simulink model "Controlador_Otimo_Aero"  (R2018a)
settings: Solver=FixedStepAuto  StartTime=0.0  StopTime=70  RelTol=1e-3  EnableMultiTasking=on
values from neighbouring files (symbols this model uses):
  C = [1 0 0 0 ... (first row only)    [Dados.m]    (also in Dados_correct.m; Function_ARE.m = D; teste.m = D)
  K1_30 = Kpi30(:,1:4)    [Dados_correct.m]
  K2_30 = Kpi30(:,5:6)    [Dados_correct.m]
  Pphi = polyfit(phi,y_phi,2)    [Pot.m]
  Pteta = polyfit(teta,y_teta,2)    [Pot.m]
undefined symbols (not defined in the file or in its folder): DiscIntNeverNeededParam, K1_130, K1_150, K1_90, K2_130, K2_150, K2_90, sigbuilder_block
libraries: arduinolib x4, simulink x2
settings Model: SimulationMode=external  ExtModeTrigDuration=2  Creator=stayn  LastModifiedBy=stayn
settings OptimizationCC: EnhancedBackFolding=on  PassReuseOutputArgsAs=Individual arguments  MaxStackSize=64  OptimizeBlockOrder=speed  DifferentSizesBufferReuse=on  OptimizationCustomize=off
settings DebuggingCC: ParameterTunabilityLossMsg=error
settings HardwareCC: ProdBitPerInt=16  ProdBitPerPointer=16  ProdBitPerSizeT=16  ProdBitPerPtrDiffT=16  ProdLargestAtomicFloat=None  ProdWordSize=8  ProdHWDeviceType=Atmel->AVR
settings SFSimCC: MATLABDynamicMemAlloc=off
settings RTWCC: SystemTargetFile=ert.tlc  HardwareBoard=Arduino Mega 2560  TLCOptions=-aInlineSetEventsForThisBaseRateFcn=TLC_FALSE -aSuppressMultiTaskScheduler=TLC_FALSE -aRateBasedStepFcn=1  TemplateMakefile=ert_default_tmf  GenerateReport=on  Toolchain=Arduino AVR  BuildConfiguration=Faster Runs  IncludeHyperlinkInReport=on  LaunchReport=on  GenerateTraceInfo=on  GenerateTraceReport=on  GenerateTraceReportSl=on  GenerateTraceReportSf=on  GenerateTraceReportEml=on
settings CodeAppCC: ForceParamTrailComments=on  IgnoreCustomStorageClasses=off  OperatorAnnotations=on  SimulinkDataObjDesc=on  SFDataObjDesc=on  InsertBlockDesc=on
settings ERTTargetCC: SupportContinuousTime=on  SupportVariableSizeSignals=on

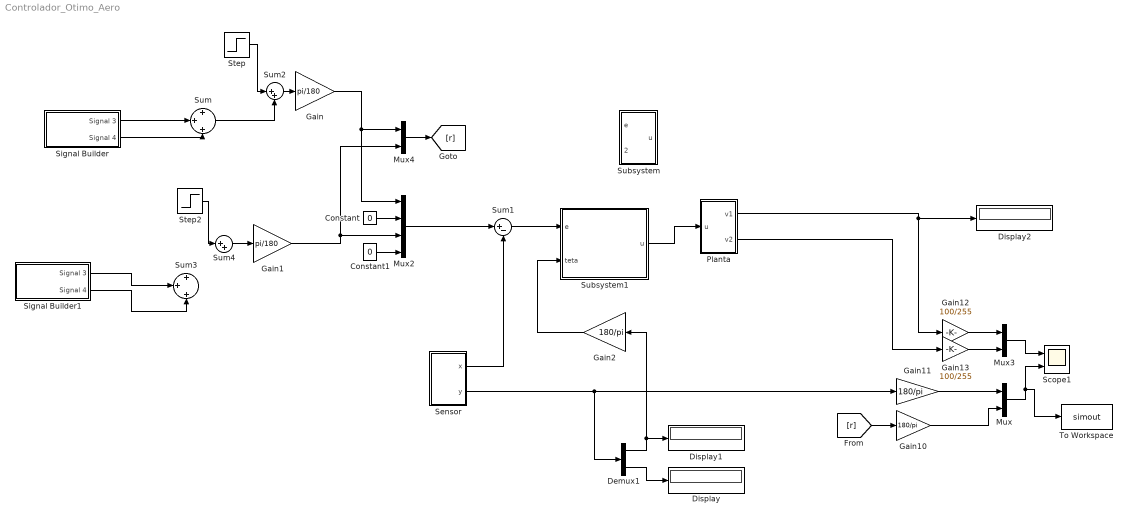
== system Controlador_Otimo_Aero ==
  Constant : Constant  Value=0
  Constant1 : Constant  Value=0
  Demux1 : Demux  Outputs=2
  Display : Display
  Display1 : Display
  Display2 : Display
  Gain : Gain  Gain=pi/180
  Gain1 : Gain  Gain=pi/180
  Gain10 : Gain  Gain=180/pi
  Gain11 : Gain  Gain=180/pi
  Gain12 : Gain  Gain=100/255
  Gain13 : Gain  Gain=100/255
  Gain2 : Gain  Gain=180/pi
  Mux : Mux  Inputs=2
  Mux2 : Mux
  Mux3 : Mux  Inputs=2
  Mux4 : Mux  Inputs=2
  Planta : Subsystem
  Scope1 : Scope  NumInputPorts=2
  Sensor : Subsystem
  Signal Builder : Subsystem  Tag=STV Subsys  LoadFcn=sigbuilder_block('load');  StartFcn=sigbuilder_block('start');  StopFcn=sigbuilder_block('stop');  ClipboardFcn=sigbuilder_block('clipboard');  mask(Sigbuilder block){tuvar=[0:10]}
      mask help: Simulink:masks:SigbuilderBlock_MD
      mask init:
      | if ~strcmp(get_param(bdroot(gcbh),'SimulationStatus'),'stopped') tuvar = sigbuilder_block('maskInit'); end
      settings: CopyFcn=sigbuilder_block('copy');  DeleteFcn=sigbuilder_block('delete');  ModelCloseFcn=sigbuilder_block('modelClose');  PreSaveFcn=sigbuilder_block('preSave');  PauseFcn=sigbuilder_block('pause');  ContinueFcn=sigbuilder_block('continue');  NameChangeFcn=sigbuilder_block('namechange');  OpenFcn=sigbuilder_block('open',[6 30 1012.5 447.75 ]);  CloseFcn=sigbuilder_block('close');
      mask Display: plot(0, 0, 100, 100,[2, 2, 32, 32, 2], [68, 8, 8, 68, 68],[32, 2], [38, 38], [32, 19, 2],[53, 60, 44], [32, 17, 17, 2],[16, 16, 31, 31]);txt = getActiveGroup(gcbh);text(2, 100, txt,'verticalAlignment', 'top');
  Signal Builder1 : Subsystem  Tag=STV Subsys  LoadFcn=sigbuilder_block('load');  StartFcn=sigbuilder_block('start');  StopFcn=sigbuilder_block('stop');  ClipboardFcn=sigbuilder_block('clipboard');  mask(Sigbuilder block){tuvar=[0:10]}
      mask help: Simulink:masks:SigbuilderBlock_MD
      mask init:
      | if ~strcmp(get_param(bdroot(gcbh),'SimulationStatus'),'stopped') tuvar = sigbuilder_block('maskInit'); end
      settings: CopyFcn=sigbuilder_block('copy');  DeleteFcn=sigbuilder_block('delete');  ModelCloseFcn=sigbuilder_block('modelClose');  PreSaveFcn=sigbuilder_block('preSave');  PauseFcn=sigbuilder_block('pause');  ContinueFcn=sigbuilder_block('continue');  NameChangeFcn=sigbuilder_block('namechange');  OpenFcn=sigbuilder_block('open',[6 30 1006.5 447.75 ]);  CloseFcn=sigbuilder_block('close');
      mask Display: plot(0, 0, 100, 100,[2, 2, 32, 32, 2], [68, 8, 8, 68, 68],[32, 2], [38, 38], [32, 19, 2],[53, 60, 44], [32, 17, 17, 2],[16, 16, 31, 31]);txt = getActiveGroup(gcbh);text(2, 100, txt,'verticalAlignment', 'top');
  Step : Step  Time=0  After=110  SampleTime=0
  Step2 : Step  After=25  SampleTime=0
  Subsystem : Subsystem
  Subsystem1 : Subsystem
  Sum : Sum  Inputs=+|+|+
  Sum1 : Sum  Inputs=|+-
  Sum2 : Sum  Inputs=|++
  Sum3 : Sum  Inputs=+|+|+
  Sum4 : Sum  Inputs=|++
  To Workspace : ToWorkspace  VariableName=simout  SampleTime=-1
      settings: Save2DSignal=2-D array (concatenate along first dimension)
  wires:
  Mux3/1 -> Scope1/1
  Mux/1 -> To Workspace/1, Scope1/2
  [r] -> Gain10/1
  Gain10/1 -> Mux/2
  Gain11/1 -> Mux/1
  Gain12/1 -> Mux3/1
  Gain13/1 -> Mux3/2
  Sum1/1 -> Subsystem1/1(e)
  Sensor/1("x ") -> Sum1/2
  Sensor/2(y) -> Demux1/1, Gain11/1
  Demux1/2 -> Display/1
  Subsystem1/1(u) -> Planta/1(u)
  Planta/1(v1) -> Display2/1, Gain12/1
  Planta/2("v2 ") -> Gain13/1
  Demux1/1 -> Display1/1, Gain2/1
  Gain2/1 -> Subsystem1/2(teta)
  Step2/1 -> Sum4/1
  Sum/1 -> Sum2/2
  Signal Builder1/1(Signal 3) -> Sum3/2
  Sum4/1 -> Gain1/1
  Signal Builder/1(Signal 3) -> Sum/2
  Signal Builder1/2(Signal 4) -> Sum3/3
  Constant1/1 -> Mux2/4
  Constant/1 -> Mux2/2
  Mux2/1 -> Sum1/1
  Mux4/1 -> [r]
  Gain1/1 -> Mux4/2, Mux2/3
  Step/1 -> Sum2/1
  Sum2/1 -> Gain/1
  Gain/1 -> Mux2/1, Mux4/1
  Signal Builder/2(Signal 4) -> Sum/3

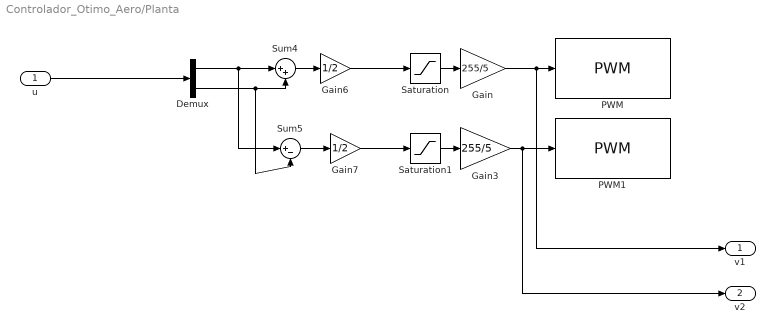
== system Controlador_Otimo_Aero/Planta ==
  u : Inport
  Demux : Demux  Outputs=2
  Gain : Gain  Gain=255/5
  Gain3 : Gain  Gain=255/5
  Gain6 : Gain  Gain=1/2
  Gain7 : Gain  Gain=1/2
  PWM : arduinolib/PWM  pinNumber=9  EnableInputFrequency=off  InitialFrequency=2000  InitialDutyCycle=0  NotificationType=None  blockPlatform=arduino
  PWM1 : arduinolib/PWM  pinNumber=8  EnableInputFrequency=off  InitialFrequency=2000  InitialDutyCycle=0  NotificationType=None  blockPlatform=arduino
  Saturation : Saturate  UpperLimit=5  LowerLimit=0
  Saturation1 : Saturate  UpperLimit=5  LowerLimit=0
  Sum4 : Sum  Inputs=|++
  Sum5 : Sum  Inputs=|+-
  v1 : Outport
  "v2 " : Outport  Port=2
  wires:
  Sum4/1 -> Gain6/1
  Demux/1 -> Sum5/1, Sum4/1
  Saturation1/1 -> Gain3/1
  Gain7/1 -> Saturation1/1
  Demux/2 -> Sum5/2, Sum4/2
  Gain/1 -> PWM/1, v1/1
  Saturation/1 -> Gain/1
  Gain6/1 -> Saturation/1
  Gain3/1 -> PWM1/1, "v2 "/1
  Sum5/1 -> Gain7/1
  u/1 -> Demux/1

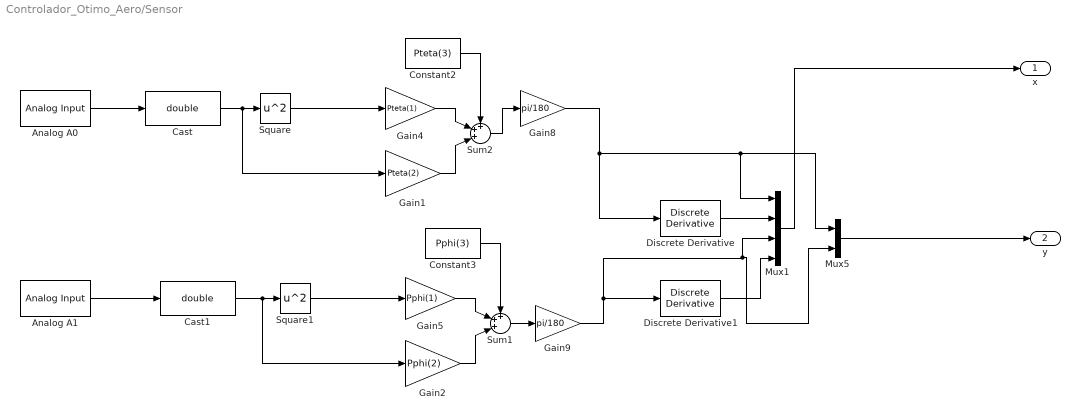
== system Controlador_Otimo_Aero/Sensor ==
  Analog A0 : arduinolib/Analog Input  pinNumber=0  ReadResultsOnly=off  ConversionTriggerSource=Software  ExternalTriggerType=uint32(0)  OutputDataType=uint16  EnableConversionCompleteNotify=off  EnableOuputStatus=off  SampleTime=-1  blockPlatform=arduino
  Analog A1 : arduinolib/Analog Input  pinNumber=1  ReadResultsOnly=off  ConversionTriggerSource=Software  ExternalTriggerType=uint32(0)  OutputDataType=uint16  EnableConversionCompleteNotify=off  EnableOuputStatus=off  SampleTime=-1  blockPlatform=arduino
  Cast : DataTypeConversion  OutDataTypeStr=double
  Cast1 : DataTypeConversion  OutDataTypeStr=double
  Constant2 : Constant  Value=Pteta(3)
  Constant3 : Constant  Value=Pphi(3)
  Discrete Derivative : simulink/Discrete/Discrete Derivative  gainval=1.0  ICPrevScaledInput=0.0  OutMin=[]  OutMax=[]  OutDataType=fixdt(1, 16)  OutScaling=2^-10  DoSatur=off
  Discrete Derivative1 : simulink/Discrete/Discrete Derivative  gainval=1.0  ICPrevScaledInput=0.0  OutMin=[]  OutMax=[]  OutDataType=fixdt(1, 16)  OutScaling=2^-10  DoSatur=off
  Gain1 : Gain  Gain=Pteta(2)
  Gain2 : Gain  Gain=Pphi(2)
  Gain4 : Gain  Gain=Pteta(1)
  Gain5 : Gain  Gain=Pphi(1)
  Gain8 : Gain  Gain=pi/180
  Gain9 : Gain  Gain=pi/180
  Mux1 : Mux
  Mux5 : Mux  Inputs=2
  Square : Math  Operator=square  SaturateOnIntegerOverflow=on
  Square1 : Math  Operator=square  SaturateOnIntegerOverflow=on
  Sum1 : Sum  Inputs=+++|
  Sum2 : Sum  Inputs=+++|
  "x " : Outport
  y : Outport  Port=2
  wires:
  Mux5/1 -> y/1
  Gain9/1 -> Discrete Derivative1/1, Mux5/2, Mux1/3
  Gain8/1 -> Mux5/1, Mux1/1, Discrete Derivative/1
  Discrete Derivative1/1 -> Mux1/4
  Mux1/1 -> "x "/1
  Discrete Derivative/1 -> Mux1/2
  Cast1/1 -> Gain2/1, Square1/1
  Square1/1 -> Gain5/1
  Sum1/1 -> Gain9/1
  Gain5/1 -> Sum1/2
  Constant3/1 -> Sum1/1
  Gain1/1 -> Sum2/3
  Analog A1/1 -> Cast1/1
  Analog A0/1 -> Cast/1
  Gain4/1 -> Sum2/2
  Cast/1 -> Gain1/1, Square/1
  Constant2/1 -> Sum2/1
  Sum2/1 -> Gain8/1
  Square/1 -> Gain4/1
  Gain2/1 -> Sum1/3

== system Controlador_Otimo_Aero/Signal Builder ==
  Demux : Demux  Tag=STV Demux  Outputs=2
  FromWs : FromWorkspace  Tag=STV FromWs  VariableName=tuvar  SampleTime=0
      SigBuilderData=|
      | common.afterFinalStr = 'Extrapolate'
      | common.sampleTime = 0
      | dataSet.timeRange = [0 100]
      | dataSet.name = 'Group 1'
      | sbobj.Groups.Name = 'Group 1'
      | sbobj.Groups.Signals(1).Name = 'Signal 3'
      | sbobj.Groups.Signals(1).XData = [0 15.1 15.1 30 30 100]
      | sbobj.Groups.Signals(1).YData = [0 0 40 40 0 0]
      | sbobj.Groups.Signals(2).Name = 'Signal 4'
      | sbobj.Groups.Signals(2).XData = [0 45 45 60 60 100]
      | sbobj.Groups.Signals(2).YData = [0 0 -71 -71 0 0]
      | sbobj.Groups.TimeRange = [0 100]
  Signal 3 : Outport  Tag=STV Outport
  Signal 4 : Outport  Tag=STV Outport  Port=2
  wires:
  FromWs/1 -> Demux/1
  Demux/1 -> Signal 3/1
  Demux/2 -> Signal 4/1

== system Controlador_Otimo_Aero/Signal Builder1 ==
  Demux : Demux  Tag=STV Demux  Outputs=2
  FromWs : FromWorkspace  Tag=STV FromWs  VariableName=tuvar  SampleTime=0
      SigBuilderData=|
      | common.afterFinalStr = 'Extrapolate'
      | common.sampleTime = 0
      | dataSet.timeRange = [0 100]
      | dataSet.name = 'Group 1'
      | sbobj.Groups.Name = 'Group 1'
      | sbobj.Groups.Signals(1).Name = 'Signal 3'
      | sbobj.Groups.Signals(1).XData = [0 15.1 15.1 30.1 30.1 100]
      | sbobj.Groups.Signals(1).YData = [0 0 15 15 0 0]
      | sbobj.Groups.Signals(2).Name = 'Signal 4'
      | sbobj.Groups.Signals(2).XData = [0 45 45 60 60 100]
      | sbobj.Groups.Signals(2).YData = [0 0 -15 -15 0 0]
      | sbobj.Groups.TimeRange = [0 100]
  Signal 3 : Outport  Tag=STV Outport
  Signal 4 : Outport  Tag=STV Outport  Port=2
  wires:
  FromWs/1 -> Demux/1
  Demux/1 -> Signal 3/1
  Demux/2 -> Signal 4/1

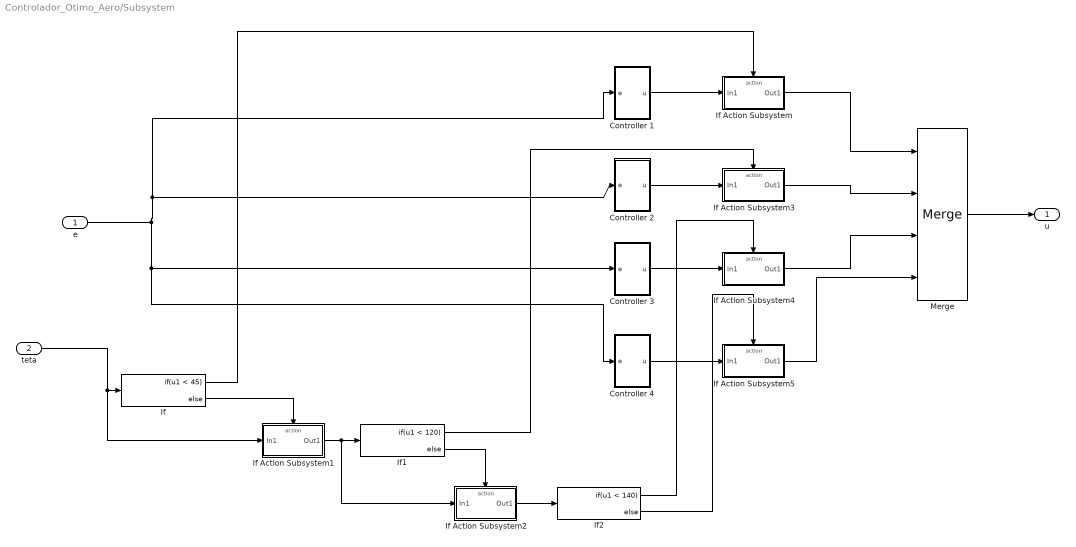
== system Controlador_Otimo_Aero/Subsystem ==
  e : Inport
  teta : Inport  Port=2
  Controller 1 : Subsystem
  Controller 2 : Subsystem
  Controller 3 : Subsystem
  Controller 4 : Subsystem
  If : If  IfExpression=u1 < 45
  If Action Subsystem : Subsystem  TreatAsAtomicUnit=on
  If Action Subsystem1 : Subsystem  TreatAsAtomicUnit=on
  If Action Subsystem2 : Subsystem  TreatAsAtomicUnit=on
  If Action Subsystem3 : Subsystem  TreatAsAtomicUnit=on
  If Action Subsystem4 : Subsystem  TreatAsAtomicUnit=on
  If Action Subsystem5 : Subsystem  TreatAsAtomicUnit=on
  If1 : If  IfExpression=u1 < 120
  If2 : If  IfExpression=u1 < 140
  Merge : Merge  Inputs=4
  u : Outport
  wires:
  Controller 3/1("u ") -> If Action Subsystem4/1(In1)
  Controller 1/1("u ") -> If Action Subsystem/1(In1)
  If2/1 -> If Action Subsystem4/Action
  e/1 -> Controller 1/1("e "), Controller 2/1("e "), Controller 4/1("e "), Controller 3/1("e ")
  If Action Subsystem4/1(Out1) -> Merge/3
  teta/1 -> If Action Subsystem1/1(In1), If/1
  If2/2 -> If Action Subsystem5/Action
  Merge/1 -> u/1
  Controller 4/1("u ") -> If Action Subsystem5/1(In1)
  If Action Subsystem/1(Out1) -> Merge/1
  If/2 -> If Action Subsystem1/Action
  Controller 2/1("u ") -> If Action Subsystem3/1(In1)
  If Action Subsystem1/1(Out1) -> If Action Subsystem2/1(In1), If1/1
  If Action Subsystem2/1(Out1) -> If2/1
  If Action Subsystem3/1(Out1) -> Merge/2
  If Action Subsystem5/1(Out1) -> Merge/4
  If/1 -> If Action Subsystem/Action
  If1/1 -> If Action Subsystem3/Action
  If1/2 -> If Action Subsystem2/Action

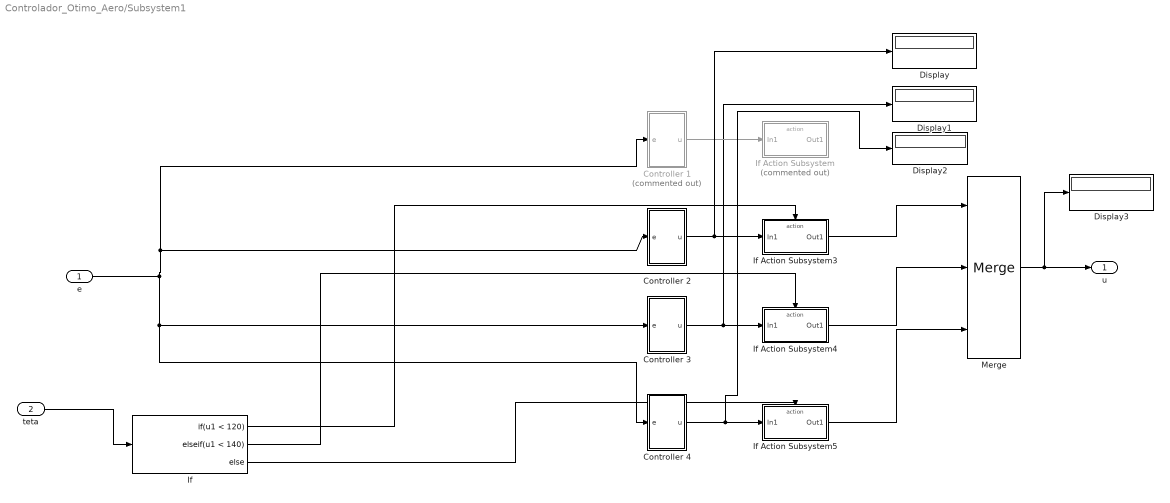
== system Controlador_Otimo_Aero/Subsystem1 ==
  e : Inport
  teta : Inport  Port=2
  Controller 1 : Subsystem  Commented=on
  Controller 2 : Subsystem
  Controller 3 : Subsystem
  Controller 4 : Subsystem
  Display{,1..3} (4 alike) : Display
  If : If  IfExpression=u1 < 120  ElseIfExpressions=u1 < 140
  If Action Subsystem : Subsystem  Commented=on  TreatAsAtomicUnit=on
  If Action Subsystem3 : Subsystem  TreatAsAtomicUnit=on
  If Action Subsystem4 : Subsystem  TreatAsAtomicUnit=on
  If Action Subsystem5 : Subsystem  TreatAsAtomicUnit=on
  Merge : Merge  Inputs=3
  u : Outport
  wires:
  Controller 3/1("u ") -> Display1/1, If Action Subsystem4/1(In1)
  Controller 1/1("u ") -> If Action Subsystem/1(In1)
  e/1 -> Controller 1/1("e "), Controller 2/1("e "), Controller 4/1("e "), Controller 3/1("e ")
  teta/1 -> If/1
  Merge/1 -> Display3/1, u/1
  Controller 4/1("u ") -> Display2/1, If Action Subsystem5/1(In1)
  Controller 2/1("u ") -> Display/1, If Action Subsystem3/1(In1)
  If/1 -> If Action Subsystem3/Action
  If Action Subsystem3/1(Out1) -> Merge/1
  If Action Subsystem4/1(Out1) -> Merge/2
  If Action Subsystem5/1(Out1) -> Merge/3
  If/3 -> If Action Subsystem5/Action
  If/2 -> If Action Subsystem4/Action

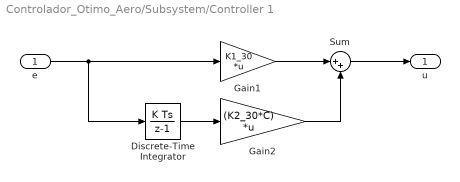
== system Controlador_Otimo_Aero/Subsystem/Controller 1 ==
  "e " : Inport
  Discrete-Time Integrator : DiscreteIntegrator  SampleTime=0.025  ICPrevOutput=DiscIntNeverNeededParam  ICPrevScaledInput=DiscIntNeverNeededParam
  Gain1 : Gain  Gain=K1_30  Multiplication=Matrix(K*u) (u vector)
  Gain2 : Gain  Gain=(K2_30*C)  Multiplication=Matrix(K*u) (u vector)
  Sum : Sum  Inputs=|++
  "u " : Outport
  wires:
  Discrete-Time Integrator/1 -> Gain2/1
  "e "/1 -> Discrete-Time Integrator/1, Gain1/1
  Gain1/1 -> Sum/1
  Gain2/1 -> Sum/2
  Sum/1 -> "u "/1

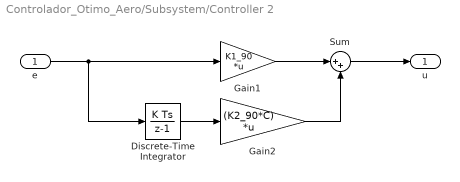
== system Controlador_Otimo_Aero/Subsystem/Controller 2 ==
  "e " : Inport
  Discrete-Time Integrator : DiscreteIntegrator  SampleTime=0.025  ICPrevOutput=DiscIntNeverNeededParam  ICPrevScaledInput=DiscIntNeverNeededParam
  Gain1 : Gain  Gain=K1_90  Multiplication=Matrix(K*u) (u vector)
  Gain2 : Gain  Gain=(K2_90*C)  Multiplication=Matrix(K*u) (u vector)
  Sum : Sum  Inputs=|++
  "u " : Outport
  wires:
  Discrete-Time Integrator/1 -> Gain2/1
  "e "/1 -> Discrete-Time Integrator/1, Gain1/1
  Gain1/1 -> Sum/1
  Gain2/1 -> Sum/2
  Sum/1 -> "u "/1

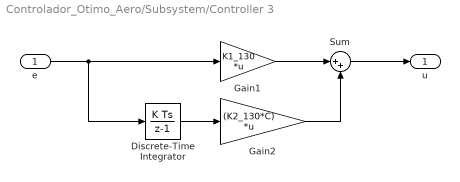
== system Controlador_Otimo_Aero/Subsystem/Controller 3 ==
  "e " : Inport
  Discrete-Time Integrator : DiscreteIntegrator  SampleTime=0.025  ICPrevOutput=DiscIntNeverNeededParam  ICPrevScaledInput=DiscIntNeverNeededParam
  Gain1 : Gain  Gain=K1_130  Multiplication=Matrix(K*u) (u vector)
  Gain2 : Gain  Gain=(K2_130*C)  Multiplication=Matrix(K*u) (u vector)
  Sum : Sum  Inputs=|++
  "u " : Outport
  wires:
  Discrete-Time Integrator/1 -> Gain2/1
  "e "/1 -> Discrete-Time Integrator/1, Gain1/1
  Gain1/1 -> Sum/1
  Gain2/1 -> Sum/2
  Sum/1 -> "u "/1

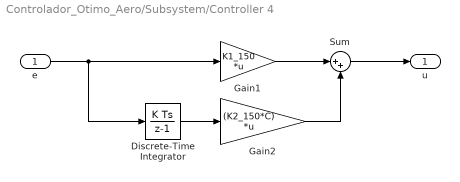
== system Controlador_Otimo_Aero/Subsystem/Controller 4 ==
  "e " : Inport
  Discrete-Time Integrator : DiscreteIntegrator  SampleTime=0.025  ICPrevOutput=DiscIntNeverNeededParam  ICPrevScaledInput=DiscIntNeverNeededParam
  Gain1 : Gain  Gain=K1_150  Multiplication=Matrix(K*u) (u vector)
  Gain2 : Gain  Gain=(K2_150*C)  Multiplication=Matrix(K*u) (u vector)
  Sum : Sum  Inputs=|++
  "u " : Outport
  wires:
  Discrete-Time Integrator/1 -> Gain2/1
  "e "/1 -> Discrete-Time Integrator/1, Gain1/1
  Gain1/1 -> Sum/1
  Gain2/1 -> Sum/2
  Sum/1 -> "u "/1

== system Controlador_Otimo_Aero/Subsystem/If Action Subsystem ==
  In1 : Inport
  Action Port : ActionPort  ActionType=then
  Out1 : Outport
  wires:
  In1/1 -> Out1/1

== system Controlador_Otimo_Aero/Subsystem/If Action Subsystem1 ==
  In1 : Inport
  Action Port : ActionPort  ActionType=else
  Out1 : Outport
  wires:
  In1/1 -> Out1/1

== system Controlador_Otimo_Aero/Subsystem/If Action Subsystem2 ==
  In1 : Inport
  Action Port : ActionPort  ActionType=else
  Out1 : Outport
  wires:
  In1/1 -> Out1/1

== system Controlador_Otimo_Aero/Subsystem/If Action Subsystem3 ==
  In1 : Inport
  Action Port : ActionPort  ActionType=then
  Out1 : Outport
  wires:
  In1/1 -> Out1/1

== system Controlador_Otimo_Aero/Subsystem/If Action Subsystem4 ==
  In1 : Inport
  Action Port : ActionPort  ActionType=then
  Out1 : Outport
  wires:
  In1/1 -> Out1/1

== system Controlador_Otimo_Aero/Subsystem/If Action Subsystem5 ==
  In1 : Inport
  Action Port : ActionPort  ActionType=else
  Out1 : Outport
  wires:
  In1/1 -> Out1/1

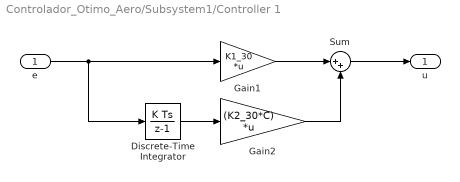
== system Controlador_Otimo_Aero/Subsystem1/Controller 1 ==
  "e " : Inport
  Discrete-Time Integrator : DiscreteIntegrator  SampleTime=0.025  ICPrevOutput=DiscIntNeverNeededParam  ICPrevScaledInput=DiscIntNeverNeededParam
  Gain1 : Gain  Gain=K1_30  Multiplication=Matrix(K*u) (u vector)
  Gain2 : Gain  Gain=(K2_30*C)  Multiplication=Matrix(K*u) (u vector)
  Sum : Sum  Inputs=|++
  "u " : Outport
  wires:
  Discrete-Time Integrator/1 -> Gain2/1
  "e "/1 -> Discrete-Time Integrator/1, Gain1/1
  Gain1/1 -> Sum/1
  Gain2/1 -> Sum/2
  Sum/1 -> "u "/1

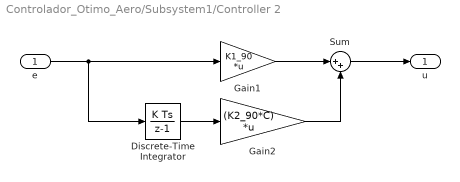
== system Controlador_Otimo_Aero/Subsystem1/Controller 2 ==
  "e " : Inport
  Discrete-Time Integrator : DiscreteIntegrator  SampleTime=0.025  ICPrevOutput=DiscIntNeverNeededParam  ICPrevScaledInput=DiscIntNeverNeededParam
  Gain1 : Gain  Gain=K1_90  Multiplication=Matrix(K*u) (u vector)
  Gain2 : Gain  Gain=(K2_90*C)  Multiplication=Matrix(K*u) (u vector)
  Sum : Sum  Inputs=|++
  "u " : Outport
  wires:
  Discrete-Time Integrator/1 -> Gain2/1
  "e "/1 -> Discrete-Time Integrator/1, Gain1/1
  Gain1/1 -> Sum/1
  Gain2/1 -> Sum/2
  Sum/1 -> "u "/1

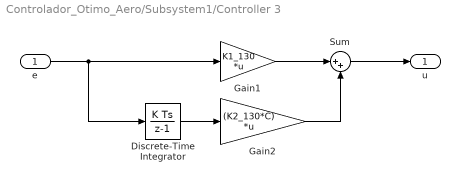
== system Controlador_Otimo_Aero/Subsystem1/Controller 3 ==
  "e " : Inport
  Discrete-Time Integrator : DiscreteIntegrator  SampleTime=0.025  ICPrevOutput=DiscIntNeverNeededParam  ICPrevScaledInput=DiscIntNeverNeededParam
  Gain1 : Gain  Gain=K1_130  Multiplication=Matrix(K*u) (u vector)
  Gain2 : Gain  Gain=(K2_130*C)  Multiplication=Matrix(K*u) (u vector)
  Sum : Sum  Inputs=|++
  "u " : Outport
  wires:
  Discrete-Time Integrator/1 -> Gain2/1
  "e "/1 -> Discrete-Time Integrator/1, Gain1/1
  Gain1/1 -> Sum/1
  Gain2/1 -> Sum/2
  Sum/1 -> "u "/1

== system Controlador_Otimo_Aero/Subsystem1/Controller 4 ==
  "e " : Inport
  Discrete-Time Integrator : DiscreteIntegrator  SampleTime=0.025  ICPrevOutput=DiscIntNeverNeededParam  ICPrevScaledInput=DiscIntNeverNeededParam
  Gain1 : Gain  Gain=K1_150  Multiplication=Matrix(K*u) (u vector)
  Gain2 : Gain  Gain=(K2_150*C)  Multiplication=Matrix(K*u) (u vector)
  Sum : Sum  Inputs=|++
  "u " : Outport
  wires:
  Discrete-Time Integrator/1 -> Gain2/1
  "e "/1 -> Discrete-Time Integrator/1, Gain1/1
  Gain1/1 -> Sum/1
  Gain2/1 -> Sum/2
  Sum/1 -> "u "/1

== system Controlador_Otimo_Aero/Subsystem1/If Action Subsystem ==
  In1 : Inport
  Action Port : ActionPort  PropagateVarSize=During execution
  Out1 : Outport
  wires:
  In1/1 -> Out1/1

== system Controlador_Otimo_Aero/Subsystem1/If Action Subsystem3 ==
  In1 : Inport
  Action Port : ActionPort  PropagateVarSize=During execution  ActionType=then
  Out1 : Outport
  wires:
  In1/1 -> Out1/1

== system Controlador_Otimo_Aero/Subsystem1/If Action Subsystem4 ==
  In1 : Inport
  Action Port : ActionPort  PropagateVarSize=During execution  ActionType=elseif
  Out1 : Outport
  wires:
  In1/1 -> Out1/1

== system Controlador_Otimo_Aero/Subsystem1/If Action Subsystem5 ==
  In1 : Inport
  Action Port : ActionPort  PropagateVarSize=During execution  ActionType=else
  Out1 : Outport
  wires:
  In1/1 -> Out1/1
